simulink model "RobotX_ss_acousticsSingle_Dock_LBskip_ODOA_T_1024_NewLidarMode"  (R2014a)
settings: Solver=FixedStepDiscrete  StartTime=0.0  StopTime=inf  FixedStep=.25  RelTol=1e-3
undefined symbols (not defined in the file): Com1, Com2, Com3, Com4, DiscIntNeverNeededParam, standard
libraries: xpcseriallib x42, simulink x19, slrtlib x7, dspmtrx3 x2, speedgoatlib x2, speedgoatlib_IO102 x1
(part 3 of 7)

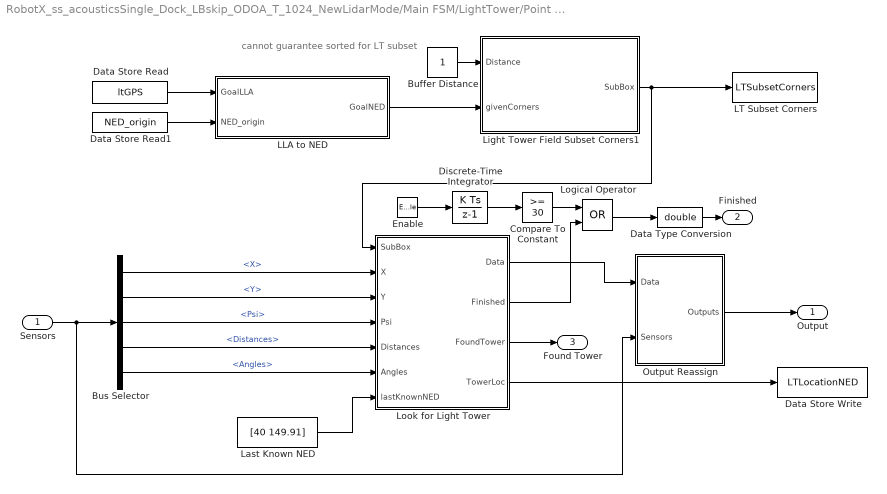
== system RobotX_ss_acousticsSingle_Dock_LBskip_ODOA_T_1024_NewLidarMode/Main FSM/LightTower/Point Toward Last Known Heading ==
  note: cannot guarantee sorted for LT subset
  Sensors : Inport
  Enable : EnablePort  ShowOutputPort=on
  Buffer Distance : Constant
  Bus Selector : BusSelector  OutputSignals=Navigation Message.Pose.X,Navigation Message.Pose.Y,Navigation Message.Pose.Psi,Lidar Data Input.Landmarks.Distances,Lidar Data Input.Landmarks.Angles
  Compare To Constant : simulink/Logic and Bit Operations/Compare To Constant  relop=>=  const=30  OutDataTypeStr=boolean
  Data Store Read : DataStoreRead  DataStoreName=ltGPS
  Data Store Read1 : DataStoreRead  DataStoreName=NED_origin
  Data Store Write : DataStoreWrite  DialogController=Simulink.DDGSource  DataStoreName=LTLocationNED
  Data Type Conversion : DataTypeConversion  OutDataTypeStr=double
  Discrete-Time Integrator : DiscreteIntegrator  SampleTime=-1  ICPrevOutput=DiscIntNeverNeededParam  ICPrevScaledInput=DiscIntNeverNeededParam
  LLA to NED : MATLAB Function  TreatAsAtomicUnit=on
  LT Subset Corners : DataStoreWrite  DataStoreName=LTSubsetCorners
  Last Known NED : Constant  Value=[40 149.91]
  Light Tower Field Subset Corners1 : MATLAB Function  TreatAsAtomicUnit=on
  Logical Operator : Logic  Operator=OR  AllPortsSameDT=off  OutDataTypeStr=boolean
  Look for Light Tower : MATLAB Function  TreatAsAtomicUnit=on
  Output Reassign : Subsystem
  Output : Outport
  Finished : Outport  Port=2
  Found Tower : Outport  Port=3
  wires:
  Output Reassign/1(Outputs) -> Output/1
  Sensors/1 -> Output Reassign/2(Sensors), Bus Selector/1
  Data Store Read/1 -> LLA to NED/1(GoalLLA)
  Data Store Read1/1 -> LLA to NED/2(NED_origin)
  LLA to NED/1(GoalNED) -> Light Tower Field Subset Corners1/2(givenCorners)
  Buffer Distance/1 -> Light Tower Field Subset Corners1/1(Distance)
  Bus Selector/1 -> Look for Light Tower/2(X)  "<X>"
  Bus Selector/2 -> Look for Light Tower/3(Y)  "<Y>"
  Bus Selector/3 -> Look for Light Tower/4(Psi)  "<Psi>"
  Bus Selector/4 -> Look for Light Tower/5(Distances)  "<Distances>"
  Bus Selector/5 -> Look for Light Tower/6(Angles)  "<Angles>"
  Light Tower Field Subset Corners1/1(SubBox) -> Look for Light Tower/1(SubBox), LT Subset Corners/1
  Look for Light Tower/1(Data) -> Output Reassign/1(Data)
  Look for Light Tower/2(Finished) -> Logical Operator/2
  Look for Light Tower/3(FoundTower) -> Found Tower/1
  Last Known NED/1 -> Look for Light Tower/7(lastKnownNED)
  Look for Light Tower/4(TowerLoc) -> Data Store Write/1
  Enable/1 -> Discrete-Time Integrator/1
  Discrete-Time Integrator/1 -> Compare To Constant/1
  Compare To Constant/1 -> Logical Operator/1
  Logical Operator/1 -> Data Type Conversion/1
  Data Type Conversion/1 -> Finished/1

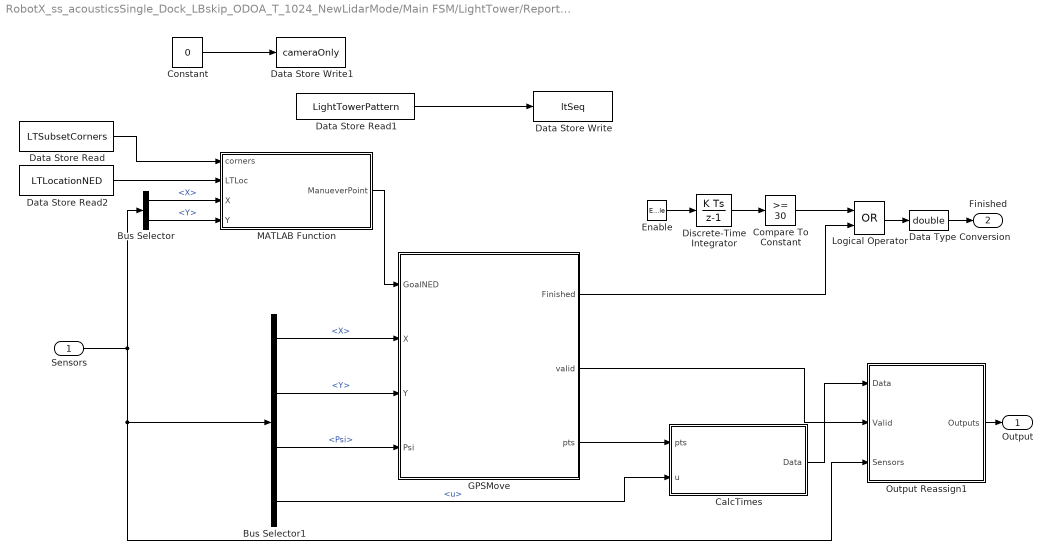
== system RobotX_ss_acousticsSingle_Dock_LBskip_ODOA_T_1024_NewLidarMode/Main FSM/LightTower/Report and Manuever Away ==
  Sensors : Inport
  Enable : EnablePort  ShowOutputPort=on
  Bus Selector : BusSelector  OutputSignals=Navigation Message.Pose.X,Navigation Message.Pose.Y
  Bus Selector1 : BusSelector  OutputSignals=Navigation Message.Pose.X,Navigation Message.Pose.Y,Navigation Message.Pose.Psi,Navigation Message.Velocity.u
  CalcTimes : MATLAB Function  TreatAsAtomicUnit=on
  Compare To Constant : simulink/Logic and Bit Operations/Compare To Constant  relop=>=  const=30  OutDataTypeStr=boolean
  Constant : Constant  Value=0
  Data Store Read : DataStoreRead  DataStoreName=LTSubsetCorners
  Data Store Read1 : DataStoreRead  DialogController=Simulink.DDGSource  DataStoreName=LightTowerPattern
  Data Store Read2 : DataStoreRead  DialogController=Simulink.DDGSource  DataStoreName=LTLocationNED
  Data Store Write : DataStoreWrite  DialogController=Simulink.DDGSource  DataStoreName=ltSeq
  Data Store Write1 : DataStoreWrite  DataStoreName=cameraOnly
  Data Type Conversion : DataTypeConversion  OutDataTypeStr=double
  Discrete-Time Integrator : DiscreteIntegrator  SampleTime=-1  ICPrevOutput=DiscIntNeverNeededParam  ICPrevScaledInput=DiscIntNeverNeededParam
  GPSMove : MATLAB Function  TreatAsAtomicUnit=on
  Logical Operator : Logic  Operator=OR  AllPortsSameDT=off  OutDataTypeStr=boolean
  MATLAB Function : MATLAB Function  TreatAsAtomicUnit=on
  Output Reassign1 : Subsystem
  Output : Outport
  Finished : Outport  Port=2
  wires:
  Output Reassign1/1(Outputs) -> Output/1
  Data Store Read/1 -> MATLAB Function/1(corners)
  Sensors/1 -> Bus Selector/1, Output Reassign1/3(Sensors), Bus Selector1/1
  Bus Selector/1 -> MATLAB Function/3(X)  "<X>"
  Bus Selector/2 -> MATLAB Function/4(Y)  "<Y>"
  GPSMove/1(Finished) -> Logical Operator/2
  GPSMove/3(pts) -> CalcTimes/1(pts)
  Bus Selector1/1 -> GPSMove/2(X)  "<X>"
  Bus Selector1/2 -> GPSMove/3(Y)  "<Y>"
  Bus Selector1/3 -> GPSMove/4(Psi)  "<Psi>"
  Bus Selector1/4 -> CalcTimes/2(u)  "<u>"
  CalcTimes/1(Data) -> Output Reassign1/1(Data)
  GPSMove/2(valid) -> Output Reassign1/2(Valid)
  MATLAB Function/1(ManueverPoint) -> GPSMove/1(GoalNED)
  Data Store Read1/1 -> Data Store Write/1
  Data Store Read2/1 -> MATLAB Function/2(LTLoc)
  Discrete-Time Integrator/1 -> Compare To Constant/1
  Enable/1 -> Discrete-Time Integrator/1
  Compare To Constant/1 -> Logical Operator/1
  Logical Operator/1 -> Data Type Conversion/1
  Data Type Conversion/1 -> Finished/1
  Constant/1 -> Data Store Write1/1

== system RobotX_ss_acousticsSingle_Dock_LBskip_ODOA_T_1024_NewLidarMode/Main FSM/LightTower/Sweep Field ==
  Sensors : Inport
  Enable : EnablePort  ShowOutputPort=on
  Bus Creator : BusCreator  Inputs=2
  Bus Selector : BusSelector  OutputSignals=Drive to Point Fin,Spin & Listen Fin
  Compare To Constant : simulink/Logic and Bit Operations/Compare To Constant  relop=>=  const=30  OutDataTypeStr=boolean
  Data Type Conversion : DataTypeConversion  OutDataTypeStr=double
  Discrete-Time Integrator : DiscreteIntegrator  SampleTime=-1  ICPrevOutput=DiscIntNeverNeededParam  ICPrevScaledInput=DiscIntNeverNeededParam
  Drive to Point : Subsystem
  Logical Operator : Logic  Operator=OR  Inputs=3  AllPortsSameDT=off  OutDataTypeStr=boolean
  Multiport Switch : MultiPortSwitch  Inputs=2
  "Spin, Listen, and Point" : Subsystem
  Sweep Field Enabler : MATLAB Function  TreatAsAtomicUnit=on
  Task Option : Subsystem
  Unit Delay : UnitDelay  SampleTime=-1
  Outputs : Outport
  Finished : Outport  Port=2
  wires:
  Drive to Point/1(Outputs) -> Multiport Switch/2
  "Spin, Listen, and Point"/1(Outputs) -> Multiport Switch/3
  Multiport Switch/1 -> Outputs/1
  Data Type Conversion/1 -> Finished/1
  Sensors/1 -> "Spin, Listen, and Point"/1(Sensors), Drive to Point/1(Sensors)
  Task Option/1(Option) -> Sweep Field Enabler/1(Sweep)
  "Spin, Listen, and Point"/2(Finished) -> Bus Creator/2  "Spin & Listen Fin"
  Sweep Field Enabler/2(drivePointEn) -> Drive to Point/Enable
  Sweep Field Enabler/1(taskSelector) -> Multiport Switch/1
  Sweep Field Enabler/3(spinListenEn) -> "Spin, Listen, and Point"/Enable
  Drive to Point/2(Finished) -> Bus Creator/1  "Drive to Point Fin"
  Bus Creator/1 -> Unit Delay/1
  "Spin, Listen, and Point"/3(Found LT) -> Logical Operator/2
  Unit Delay/1 -> Bus Selector/1
  Bus Selector/1 -> Sweep Field Enabler/2(drivePointFin)  "<Drive to Point Fin>"
  Bus Selector/2 -> Sweep Field Enabler/3(spinFin)  "<Spin & Listen Fin>"
  Drive to Point/3(Found LT) -> Logical Operator/1
  Logical Operator/1 -> Data Type Conversion/1
  Discrete-Time Integrator/1 -> Compare To Constant/1
  Enable/1 -> Discrete-Time Integrator/1
  Compare To Constant/1 -> Logical Operator/3

== system RobotX_ss_acousticsSingle_Dock_LBskip_ODOA_T_1024_NewLidarMode/Main FSM/LightTower/Turn For Approach1  ==
  note: Signal
  Sensors : Inport
  Enable : EnablePort  ShowOutputPort=on
  Bus Selector : BusSelector  OutputSignals=Navigation Message.Pose.X,Navigation Message.Pose.Y
  Compare To Constant : simulink/Logic and Bit Operations/Compare To Constant  relop=>=  const=30  OutDataTypeStr=boolean
  Data Type Conversion : DataTypeConversion  OutDataTypeStr=double
  Discrete-Time Integrator : DiscreteIntegrator  SampleTime=-1  ICPrevOutput=DiscIntNeverNeededParam  ICPrevScaledInput=DiscIntNeverNeededParam
  LTLoc : DataStoreRead  DialogController=Simulink.DDGSource  DataStoreName=LTLocationNED
  MATLAB1 Function : MATLAB Function  TreatAsAtomicUnit=on
  Output Heirarchy : Subsystem
  Outputs : Outport
  Finished : Outport  Port=2
  wires:
  Discrete-Time Integrator/1 -> Compare To Constant/1
  Enable/1 -> Discrete-Time Integrator/1
  Compare To Constant/1 -> Data Type Conversion/1
  Data Type Conversion/1 -> Finished/1
  Sensors/1 -> Bus Selector/1, Output Heirarchy/2(Sensors)
  MATLAB1 Function/1(Data) -> Output Heirarchy/1(Data)
  Output Heirarchy/1(Outputs) -> Outputs/1
  Bus Selector/2 -> MATLAB1 Function/3(Y)  "<Y>"
  Bus Selector/1 -> MATLAB1 Function/2(X)  "<X>"
  LTLoc/1 -> MATLAB1 Function/1(LTLoc)

== system RobotX_ss_acousticsSingle_Dock_LBskip_ODOA_T_1024_NewLidarMode/Main FSM/LightTower/Turn For Sweep ==
  note: Signal
  Sensors : Inport
  Enable : EnablePort  ShowOutputPort=on
  Bus Selector : BusSelector  OutputSignals=Navigation Message.Pose.X,Navigation Message.Pose.Y
  Compare To Constant : simulink/Logic and Bit Operations/Compare To Constant  relop=>=  const=30  OutDataTypeStr=boolean
  Data Store Read : DataStoreRead  DataStoreName=ltGPS
  Data Store Read1 : DataStoreRead  DataStoreName=NED_origin
  Data Type Conversion : DataTypeConversion  OutDataTypeStr=double
  Discrete-Time Integrator : DiscreteIntegrator  SampleTime=-1  ICPrevOutput=DiscIntNeverNeededParam  ICPrevScaledInput=DiscIntNeverNeededParam
  LLA to NED : MATLAB Function  TreatAsAtomicUnit=on
  MATLAB Function : MATLAB Function  TreatAsAtomicUnit=on
  Output Heirarchy : Subsystem
  Outputs : Outport
  Finished : Outport  Port=2
  wires:
  Discrete-Time Integrator/1 -> Compare To Constant/1
  Enable/1 -> Discrete-Time Integrator/1
  Compare To Constant/1 -> Data Type Conversion/1
  Data Type Conversion/1 -> Finished/1
  Sensors/1 -> Bus Selector/1, Output Heirarchy/2(Sensors)
  MATLAB Function/1(Data) -> Output Heirarchy/1(Data)
  Output Heirarchy/1(Outputs) -> Outputs/1
  Bus Selector/2 -> MATLAB Function/3(Y)  "<Y>"
  Bus Selector/1 -> MATLAB Function/2(X)  "<X>"
  Data Store Read/1 -> LLA to NED/1(GoalLLA)
  Data Store Read1/1 -> LLA to NED/2(NED_origin)
  LLA to NED/1(GoalNED) -> MATLAB Function/1(ltPTS)

== system RobotX_ss_acousticsSingle_Dock_LBskip_ODOA_T_1024_NewLidarMode/Main FSM/LightTower/Wait for Sequence ==
  Sensors : Inport
  Enable : EnablePort  ShowOutputPort=on
  Bus Selector1 : BusSelector  OutputSignals=Lidar Data Input.Color data.Color
  Constant : Constant
  Data Store Read : DataStoreRead  DataStoreName=holdPose
  Data Store Write : DataStoreWrite  DataStoreName=LightTowerPattern
  Data Store Write1 : DataStoreWrite  DataStoreName=cameraOnly
  Discrete-Time Integrator : DiscreteIntegrator  SampleTime=-1  ICPrevOutput=DiscIntNeverNeededParam  ICPrevScaledInput=DiscIntNeverNeededParam
  MATLAB Function : MATLAB Function  TreatAsAtomicUnit=on
  MATLAB Function1 : MATLAB Function  TreatAsAtomicUnit=on
  Output Reassign1 : Subsystem
  Output : Outport
  Finished : Outport  Port=2
  wires:
  Sensors/1 -> Bus Selector1/1, Output Reassign1/2(Sensors)
  Output Reassign1/1(Outputs) -> Output/1
  MATLAB Function/1(Data) -> Output Reassign1/1(Data)
  MATLAB Function1/2(Pattern) -> Data Store Write/1
  Bus Selector1/1 -> MATLAB Function1/2(visionData)  "<Color>"
  Enable/1 -> Discrete-Time Integrator/1
  Discrete-Time Integrator/1 -> MATLAB Function1/1(time)
  MATLAB Function1/1(Finished) -> Finished/1
  Data Store Read/1 -> MATLAB Function/1(holdPose)
  Constant/1 -> Data Store Write1/1

== system RobotX_ss_acousticsSingle_Dock_LBskip_ODOA_T_1024_NewLidarMode/Main FSM/ODOA/Dodge ==
  Sensors : Inport
  Enable : EnablePort  ShowOutputPort=on
  Bus Selector : BusSelector  OutputSignals=Navigation Message.Pose.X,Navigation Message.Pose.Y,Navigation Message.Pose.Psi,Lidar Data Input.Landmarks.Distances,Lidar Data Input.Landmarks.Angles,Navigation Message.Velocity.u
  CalcTimes : MATLAB Function  TreatAsAtomicUnit=on
  Constant : Constant  Value=0
  Data Store Write : DataStoreWrite  DataStoreName=dodgeStart
  Discrete-Time Integrator : DiscreteIntegrator  SampleTime=-1  ICPrevOutput=DiscIntNeverNeededParam  ICPrevScaledInput=DiscIntNeverNeededParam
  Dodge : MATLAB Function  TreatAsAtomicUnit=on
  Nav Logic : MATLAB Function  Commented=on  TreatAsAtomicUnit=on
  Output Reassign : Subsystem
  Unit Delay1 : UnitDelay  InitialCondition=1  SampleTime=-1
  Outputs : Outport
  Dodge Incomplete : Outport  Port=2
  wires:
  Sensors/1 -> Output Reassign/3(Sensors), Bus Selector/1
  Enable/1 -> Discrete-Time Integrator/1
  Discrete-Time Integrator/1 -> Dodge/1(time)
  Constant/1 -> Unit Delay1/1
  Unit Delay1/1 -> Data Store Write/1
  Output Reassign/1(Outputs) -> Outputs/1
  Bus Selector/3 -> Dodge/4(Psi)  "<Psi>"
  Bus Selector/5 -> Dodge/6(Angles)  "<Angles>"
  Bus Selector/1 -> Dodge/2(X)  "<X>"
  Bus Selector/2 -> Dodge/3(Y)  "<Y>"
  Bus Selector/4 -> Dodge/5(Dist)  "<Distances>"
  Dodge/3(pts) -> CalcTimes/1(pts)
  Bus Selector/6 -> CalcTimes/2(u)  "<u>"
  Dodge/2(Valid) -> Output Reassign/1(Vaild)
  CalcTimes/1(Data) -> Output Reassign/2(Data)
  Dodge/1(dodgeIncomplete) -> Dodge Incomplete/1

== system RobotX_ss_acousticsSingle_Dock_LBskip_ODOA_T_1024_NewLidarMode/Main FSM/ODOA/Entry Gate ==
  Sensors : Inport
  Enable : EnablePort
  Bus Creator : BusCreator  Inputs=2
  Bus Selector : BusSelector  OutputSignals=Start Fin,Align Fin
  Entry Gate Align : Subsystem  TreatAsAtomicUnit=on
  Entry Gate Enabler : MATLAB Function  TreatAsAtomicUnit=on
  Entry Gate Through : Subsystem
  GPS Move : Subsystem
  Multiport Switch : MultiPortSwitch
  Unit Delay : UnitDelay  SampleTime=-1
  Outputs : Outport
  Finished : Outport  Port=2
  wires:
  Multiport Switch/1 -> Outputs/1
  Entry Gate Enabler/3(AlignEn) -> Entry Gate Align/Enable
  Sensors/1 -> GPS Move/1(Sensors), Entry Gate Through/1(Sensors), Entry Gate Align/1(Sensors)
  Entry Gate Through/2(Finished) -> Finished/1
  Entry Gate Enabler/4(ThroughEn) -> Entry Gate Through/Enable
  Unit Delay/1 -> Bus Selector/1
  Entry Gate Through/1(Outputs) -> Multiport Switch/4
  Entry Gate Enabler/1(TaskSelector) -> Multiport Switch/1
  Entry Gate Enabler/2(StartEn) -> GPS Move/Enable
  GPS Move/2(Finished) -> Bus Creator/1  "Start Fin"
  Entry Gate Align/2(Finished) -> Bus Creator/2  "Align Fin"
  Entry Gate Align/1(Outputs) -> Multiport Switch/3
  GPS Move/1(Outputs) -> Multiport Switch/2
  Bus Creator/1 -> Unit Delay/1
  Bus Selector/2 -> Entry Gate Enabler/2(AlignFin)  "<Align Fin>"
  Bus Selector/1 -> Entry Gate Enabler/1(StartFin)  "<Start Fin>"

== system RobotX_ss_acousticsSingle_Dock_LBskip_ODOA_T_1024_NewLidarMode/Main FSM/ODOA/Exit Gate ==
  Sensors : Inport
  Enable : EnablePort
  Exit Gate Align : Subsystem  TreatAsAtomicUnit=on
  Exit Gate Through : Subsystem
  Multiport Switch : MultiPortSwitch  Inputs=2
  Unit Delay : UnitDelay  SampleTime=-1
  exit Gate Enabler : MATLAB Function  TreatAsAtomicUnit=on
  Outputs : Outport
  Finished : Outport  Port=2
  wires:
  Multiport Switch/1 -> Outputs/1
  exit Gate Enabler/2(AlignEn) -> Exit Gate Align/Enable
  Sensors/1 -> Exit Gate Through/1(Sensors), Exit Gate Align/1(Sensors)
  Exit Gate Through/2(Finished) -> Finished/1
  exit Gate Enabler/3(ThroughEn) -> Exit Gate Through/Enable
  Exit Gate Through/1(Outputs) -> Multiport Switch/3
  exit Gate Enabler/1(TaskSelector) -> Multiport Switch/1
  Exit Gate Align/2(Finished) -> Unit Delay/1  "Align Fin"
  Exit Gate Align/1(Outputs) -> Multiport Switch/2
  Unit Delay/1 -> exit Gate Enabler/1(AlignFin)

== system RobotX_ss_acousticsSingle_Dock_LBskip_ODOA_T_1024_NewLidarMode/Main FSM/ODOA/GPS Beeline ==
  Sensors : Inport
  Enable : EnablePort
  Bus Selector : BusSelector  OutputSignals=Navigation Message.Pose.X,Navigation Message.Pose.Y,Navigation Message.Pose.Psi,Lidar Data Input.Landmarks.Distances,Navigation Message.Velocity.u
  CalcTimes : MATLAB Function  TreatAsAtomicUnit=on
  Data Store Read : DataStoreRead  DataStoreName=ExitGateNED
  Data Store Read1 : DataStoreRead  DataStoreName=ODOAexit
  Data Store Write : DataStoreWrite  DataStoreName=dodgeStart
  GPSMove : MATLAB Function  TreatAsAtomicUnit=on
  MATLAB Function1 : MATLAB Function  TreatAsAtomicUnit=on
  Output Reassign : Subsystem
  Unit Delay1 : UnitDelay  SampleTime=-1
  Outputs : Outport
  Finished : Outport  Port=2
  wires:
  GPSMove/4(pts) -> CalcTimes/1(pts)
  Sensors/1 -> Output Reassign/3(Sensors), Bus Selector/1
  Bus Selector/1 -> GPSMove/2(X)  "<X>"
  Bus Selector/2 -> GPSMove/3(Y)  "<Y>"
  Bus Selector/3 -> GPSMove/4(Psi)  "<Psi>"
  Bus Selector/5 -> CalcTimes/2(u)  "<u>"
  GPSMove/2(Finished) -> Finished/1
  Output Reassign/1(Outputs) -> Outputs/1
  CalcTimes/1(Data) -> Output Reassign/2(Data)
  GPSMove/3(valid) -> Output Reassign/1(Vaild)
  MATLAB Function1/1(exitGPS) -> GPSMove/1(GoalNED)
  Data Store Read1/1 -> MATLAB Function1/2(gateNumber)
  Data Store Read/1 -> MATLAB Function1/1(ExitGateGPS)
  Unit Delay1/1 -> Data Store Write/1
  Bus Selector/4 -> GPSMove/5(Distances)  "<Distances>"
  GPSMove/1(dodgeStart) -> Unit Delay1/1

== system RobotX_ss_acousticsSingle_Dock_LBskip_ODOA_T_1024_NewLidarMode/Main FSM/RCHold/Direct Control ==
  Sensors : Inport
  Acoustic Active : Constant  Value=0
  Bus Creator2 : BusCreator  Inputs=3
  Bus Creator3 : BusCreator  Inputs=3
  Bus Creator4 : BusCreator  Inputs=2
  Constant : Constant
  Constant1 : Constant  Value=2
  Constant2 : Constant  Value=zeros(24,1)
  Lidar Mode : Constant  Value=3
  Outputs : Outport
  wires:
  Sensors/1 -> Bus Creator4/2  "Sensors"
  Bus Creator4/1 -> Outputs/1  "Output Signals"
  Bus Creator2/1 -> Bus Creator3/1  "Navigation Outputs"
  Acoustic Active/1 -> Bus Creator3/2  "Acoustic Active"
  Lidar Mode/1 -> Bus Creator3/3  "Lidar Mode"
  Bus Creator3/1 -> Bus Creator4/1  "Outputs"
  Constant/1 -> Bus Creator2/1  "Valid"
  Constant1/1 -> Bus Creator2/2  "Control Mode"
  Constant2/1 -> Bus Creator2/3  "Data"

== system RobotX_ss_acousticsSingle_Dock_LBskip_ODOA_T_1024_NewLidarMode/Main FSM/Start//Speedgate/Aim ==
  note: Signal
  Sensors : Inport
  Enable : EnablePort  ShowOutputPort=on
  Compare To Constant : simulink/Logic and Bit Operations/Compare To Constant  relop=>=  const=30  OutDataTypeStr=boolean
  Data Store Read : DataStoreRead  DataStoreName=ssHeldHeading
  Data Store Read1 : DataStoreRead  Commented=on  DataStoreName=startGPS
  Data Store Read2 : DataStoreRead  Commented=on  DataStoreName=NED_origin
  Data Store Read3 : DataStoreRead  DataStoreName=startNED
  Data Type Conversion : DataTypeConversion  OutDataTypeStr=double
  Discrete-Time Integrator : DiscreteIntegrator  SampleTime=-1  ICPrevOutput=DiscIntNeverNeededParam  ICPrevScaledInput=DiscIntNeverNeededParam
  LLA to NED : MATLAB Function  Commented=on  TreatAsAtomicUnit=on
  MATLAB Function : MATLAB Function  TreatAsAtomicUnit=on
  Output Heirarchy : Subsystem
  Outputs : Outport
  Finished : Outport  Port=2
  wires:
  Discrete-Time Integrator/1 -> Compare To Constant/1
  Enable/1 -> Discrete-Time Integrator/1
  Compare To Constant/1 -> Data Type Conversion/1
  Data Type Conversion/1 -> Finished/1
  Sensors/1 -> Output Heirarchy/2(Sensors)
  MATLAB Function/1(Data) -> Output Heirarchy/1(Data)
  Output Heirarchy/1(Outputs) -> Outputs/1
  Data Store Read/1 -> MATLAB Function/1(ssHeldHeading)
  LLA to NED/1(GoalNED) -> ?
  Data Store Read2/1 -> LLA to NED/2(NED_origin)
  Data Store Read1/1 -> LLA to NED/1(LLA)
  Data Store Read3/1 -> MATLAB Function/2(ssGateNED)

== system RobotX_ss_acousticsSingle_Dock_LBskip_ODOA_T_1024_NewLidarMode/Main FSM/Start//Speedgate/Dead Reckon ==
  note: Through Gate
  Sensors : Inport
  Enable : EnablePort
  Bus Selector : BusSelector  OutputSignals=Navigation Message.Pose.X,Navigation Message.Pose.Y,Navigation Message.Velocity.u
  Calculate Times : MATLAB Function  TreatAsAtomicUnit=on
  Data Store Read : DataStoreRead  DataStoreName=ssHeldHeading
  Gate : MATLAB Function  TreatAsAtomicUnit=on
  Output Reassign : Subsystem
  sglength : Constant  Value=15
  Outputs : Outport
  Finished : Outport  Port=2
  wires:
  Output Reassign/1(Outputs) -> Outputs/1
  Gate/1(Finished) -> Finished/1
  Sensors/1 -> Output Reassign/3(Sensors), Bus Selector/1
  Bus Selector/2 -> Gate/4(Y)  "<Y>"
  Bus Selector/1 -> Gate/3(X)  "<X>"
  Bus Selector/3 -> Calculate Times/2(u)  "<u>"
  Gate/3(pts) -> Calculate Times/1(pts)
  Calculate Times/1(Data) -> Output Reassign/2(Data)
  Gate/2(Valid) -> Output Reassign/1(Vaild)
  Data Store Read/1 -> Gate/2(ssHeldHeading)
  sglength/1 -> Gate/1(sglength)

== system RobotX_ss_acousticsSingle_Dock_LBskip_ODOA_T_1024_NewLidarMode/Main FSM/Start//Speedgate/GPS Move ==
  Sensors : Inport
  Enable : EnablePort
  Bus Selector : BusSelector  OutputSignals=Navigation Message.Pose.X,Navigation Message.Pose.Y,Navigation Message.Pose.Psi,Navigation Message.Velocity.u
  CalcTimes : MATLAB Function  TreatAsAtomicUnit=on
  Data Store Read1 : DataStoreRead  Commented=on  DataStoreName=startGPS
  Data Store Read2 : DataStoreRead  Commented=on  DataStoreName=NED_origin
  Data Store Read3 : DataStoreRead  DataStoreName=startNED
  GPSMove : MATLAB Function  TreatAsAtomicUnit=on
  LLA to NED : MATLAB Function  Commented=on  TreatAsAtomicUnit=on
  Output Reassign : Subsystem
  Outputs : Outport
  Finished : Outport  Port=2
  wires:
  GPSMove/3(pts) -> CalcTimes/1(pts)
  Sensors/1 -> Output Reassign/3(Sensors), Bus Selector/1
  Bus Selector/1 -> GPSMove/2(X)  "<X>"
  Bus Selector/2 -> GPSMove/3(Y)  "<Y>"
  Bus Selector/3 -> GPSMove/4(Psi)  "<Psi>"
  Bus Selector/4 -> CalcTimes/2(u)  "<u>"
  GPSMove/1(Finished) -> Finished/1
  Output Reassign/1(Outputs) -> Outputs/1
  CalcTimes/1(Data) -> Output Reassign/2(Data)
  GPSMove/2(valid) -> Output Reassign/1(Vaild)
  LLA to NED/1(GoalNED) -> ?
  Data Store Read3/1 -> GPSMove/1(GoalNED)
  Data Store Read2/1 -> LLA to NED/2(NED_origin)
  Data Store Read1/1 -> LLA to NED/1(LLA)

== system RobotX_ss_acousticsSingle_Dock_LBskip_ODOA_T_1024_NewLidarMode/Main FSM/Termination/Output Reassign ==
  Vaild : Inport
  Data : Inport  Port=2
  Sensors : Inport  Port=3
  Acoustic Active : Constant  Value=0
  Bus Creator2 : BusCreator  Inputs=3
  Bus Creator3 : BusCreator  Inputs=3
  Bus Creator5 : BusCreator  Inputs=2
  Constant3 : Constant  Value=0
  Lidar Mode : Constant  Value=0
  Outputs : Outport
  wires:
  Sensors/1 -> Bus Creator5/2  "Sensors"
  Bus Creator5/1 -> Outputs/1  "Output Signals"
  Vaild/1 -> Bus Creator2/1  "Valid"
  Constant3/1 -> Bus Creator2/2  "Control Mode"
  Data/1 -> Bus Creator2/3  "Data"
  Bus Creator2/1 -> Bus Creator3/1  "Navigation Outputs"
  Acoustic Active/1 -> Bus Creator3/2  "Acoustic Active"
  Lidar Mode/1 -> Bus Creator3/3  "Lidar Mode"
  Bus Creator3/1 -> Bus Creator5/1  "Outputs"

== system RobotX_ss_acousticsSingle_Dock_LBskip_ODOA_T_1024_NewLidarMode/Sensors/1020 Comms/ Raspberry Pi LCM (Acoustic) ==
  LCM Input : Inport
  ASCII Decode 6 : xpcseriallib/ASCII Decode   format=Deploy:%1u, Elapsed:%g, Bearing1:%g Bearing2:%g \r\n  nvars=4  vartypes={}
  Bus Creator : BusCreator  Inputs=2
  Bus Creator1 : BusCreator  Inputs=3
  FIFO ASCII read 1 : xpcseriallib/FIFO ASCII read   header={'Deploy:'}  term=[13 10]  hold=Zero output if no new data  enable=off  maxsize=1024  outputtype=8 bit uint null terminated  sampletime=-1
  LCM Output : Outport
  wires:
  LCM Input/1 -> FIFO ASCII read 1/1
  FIFO ASCII read 1/1 -> ASCII Decode 6/1
  ASCII Decode 6/3 -> Bus Creator/1  "Horizontal Bearing"
  ASCII Decode 6/4 -> Bus Creator/2  "Vertical Bearing"
  Bus Creator/1 -> Bus Creator1/3  "Bearings"
  ASCII Decode 6/2 -> Bus Creator1/2  "Elapsed Time"
  ASCII Decode 6/1 -> Bus Creator1/1  "Deployed"
  Bus Creator1/1 -> LCM Output/1  "Acoustic Message"

== system RobotX_ss_acousticsSingle_Dock_LBskip_ODOA_T_1024_NewLidarMode/Sensors/1020 Comms/ Raspberry Pi LCM (Navigation and Acoustics) ==
  LCM Input : Inport
  ASCII Decode 6 : xpcseriallib/ASCII Decode   format=P1:%f P2:%f P3:%f V1:%f V2:%f V3:%f E1:%f E2:%f E3:%f Pt1:%f Pt2:%f St1:%f St2:%f Start:%f Elapsed:%f RC:%d Deploy:%u, Elapsed:%g, Bearing1:%g Bearing2:%g \r\n  nvars=22  vartypes={}
  Bus Creator{,5..7} (4 alike) : BusCreator  Inputs=2
  Bus Creator{1..3,8} (4 alike) : BusCreator  Inputs=3
  Bus Creator4 : BusCreator  Inputs=9
  Data Type Conversion : DataTypeConversion  OutDataTypeStr=double
  FIFO ASCII read 1 : xpcseriallib/FIFO ASCII read   header={'P1:'}  term=[13 10]  hold=Zero output if no new data  enable=off  maxsize=2048  outputtype=8 bit uint null terminated  sampletime=-1
  Navigation LCM : Outport
  Acoustic LCM : Outport  Port=2
  wires:
  LCM Input/1 -> FIFO ASCII read 1/1
  FIFO ASCII read 1/1 -> ASCII Decode 6/1
  Bus Creator4/1 -> Navigation LCM/1  "Navigation Message"
  ASCII Decode 6/1 -> Bus Creator1/1  "X"
  ASCII Decode 6/2 -> Bus Creator1/2  "Y"
  ASCII Decode 6/3 -> Bus Creator1/3  "Psi"
  Bus Creator1/1 -> Bus Creator4/1  "Pose"
  ASCII Decode 6/4 -> Bus Creator2/1  "u"
  ASCII Decode 6/5 -> Bus Creator2/2  "v"
  Bus Creator2/1 -> Bus Creator4/2  "Velocity"
  ASCII Decode 6/7 -> Bus Creator3/1  "Roll"
  ASCII Decode 6/8 -> Bus Creator3/2  "Pitch"
  ASCII Decode 6/9 -> Bus Creator3/3  "Yaw"
  Bus Creator3/1 -> Bus Creator4/3  "Euler"
  Bus Creator5/1 -> Bus Creator4/5  "Port"
  Bus Creator6/1 -> Bus Creator4/6  "Stbd"
  ASCII Decode 6/14 -> Bus Creator6/1  "StThrust"
  ASCII Decode 6/15 -> Bus Creator6/2  "StAzimuth"
  ASCII Decode 6/12 -> Bus Creator5/1  "PtThrust"
  ASCII Decode 6/13 -> Bus Creator5/2  "PtAzimuth"
  ASCII Decode 6/16 -> Bus Creator4/7  "Start"
  ASCII Decode 6/17 -> Bus Creator4/8  "Elapsed"
  ASCII Decode 6/18 -> Data Type Conversion/1  "On/Off/RC/Auto"
  Data Type Conversion/1 -> Bus Creator4/9  "On/Off/RC/Auto"
  ASCII Decode 6/6 -> Bus Creator2/3  "r"
  ASCII Decode 6/10 -> Bus Creator7/1  "Lat"
  ASCII Decode 6/11 -> Bus Creator7/2  "Long"
  Bus Creator7/1 -> Bus Creator4/4  "GPS (LLA)"
  ASCII Decode 6/21 -> Bus Creator/1  "Horizontal Bearing"
  ASCII Decode 6/22 -> Bus Creator/2  "Vertical Bearing"
  Bus Creator/1 -> Bus Creator8/3  "Bearings"
  ASCII Decode 6/20 -> Bus Creator8/2  "Elapsed Time"
  ASCII Decode 6/19 -> Bus Creator8/1  "Deployed"
  Bus Creator8/1 -> Acoustic LCM/1  "Acoustic Message"

== matlab function RobotX_ss_acousticsSingle_Dock_LBskip_ODOA_T_1024_NewLidarMode/Main FSM/Acoustic Single Point FSM/Move/GPSMove ==
  data: GoalNED input; X input; Finished output; valid output; Y input; Psi input; pts output
function [Finished,valid,pts] = GPSmove(GoalNED,X,Y,Psi)
%Written by Dylan DeGaetano on September 1, 2014
%Last edited by: Anderson Lebbad
%
%This function will go to a given NED cooridnate, last edit changed the
%goal pt and variable names

persistent Sample
if isempty(Sample)
Sample = 0;
end
Finished = 0;
pts = zeros(8,2);
%$Distance to object in meters
if Sample >= 100
    Sample = 0;
end

if Sample == 0
    pts(1,1) = X+5*cos(Psi*pi/180);
    pts(1,2) = Y+5*sin(Psi*pi/180);
    pts(8,1) = GoalNED(1,1);
    pts(8,2) = GoalNED(1,2);
    pts(2,:) = pts(1,:) +(1*(GoalNED-pts(1,:))/7);
    pts(3,:) = pts(1,:) +(2*(GoalNED-pts(1,:))/7);
    pts(4,:) = pts(1,:) +(3*(GoalNED-pts(1,:))/7);
    pts(5,:) = pts(1,:) +(4*(GoalNED-pts(1,:))/7);
    pts(6,:) = pts(1,:) +(5*(GoalNED-pts(1,:))/7);
    pts(7,:) = pts(1,:) +(6*(GoalNED-pts(1,:))/7);
    Sample = 1; 
    valid = 1;
    
else 
    range = sqrt(sum((GoalNED - [X Y]).^2));
    if range <= 5
        Finished = 1;
    end
    valid = 0;
    Sample = Sample + 1;
end

== matlab function RobotX_ss_acousticsSingle_Dock_LBskip_ODOA_T_1024_NewLidarMode/Main FSM/LightTower/Point Toward Last Known Heading/LLA to NED ==
  data: GoalLLA input; GoalNED output; NED_origin input
function GoalNED = LLA2NEDfun(GoalLLA,NED_origin)
%Written by Anderson Lebbad on September 20, 2014
%Last edited by:
%
%This function converts a target Latitude, Longitude, Altitude (LLA) point
%into North, East, Down (NED) coordinates
GoalNED = zeros(size(GoalLLA));
for i = 1:size(GoalLLA,1)
    %First convert to earth centered, earth fixed frame
    GoalECEF = lla2ecef([GoalLLA(1)*(pi/180), GoalLLA(2)*(pi/180), 0]');
    %Then convert from ECEF to North East Down
    GoalNEDvect = ecef2ned([NED_origin(1)*(pi/180),NED_origin(2)*(pi/180)],GoalECEF);
    GoalNED(i,:) = GoalNEDvect(1:2)';
end

end

function x_ecef = lla2ecef(x_lla)
% LLE2ECEF: Converts from geodetic latitude, longitude, and altitude to earth-centered earth-fixed Cartesian coordinates
% INPUT: latitude phi (rad), longitude lambda (rad), altitude h (m)
% OUTPUT: [x, y, z]' (m) earth-centered earth-fixed Cartesian coordinates
    a = 6378137; % equatorial radius of ellipsoid (semi-major axis) (m)
    b = 6356752; % polar axis radius of ellipsoid (semi-minor axis) (m)

    phi = x_lla(1);
    lambda = x_lla(2);
    h = x_lla(3);
    
    % auxiliar quantities f, e, and N
    f = (a-b)/a;
    e = f*(2-f);
    N = a/sqrt(1-(e*sin(phi))^2);
    x_ecef = [(N+h)*cos(phi)*cos(lambda); (N+h)*cos(phi)*sin(lambda); (N*(1-e^2)+h)*sin(phi)];
end

function [x_ned] = ecef2ned(ned_lla, x_ecef)
% ECEF2NED Converts from earth-centered, earth-fixed Cartesian coordinates to tangent plane
% INPUT:
% 1) x_ecef=[x,y,z]' (m) earth-centered, earth-fixed Cartesian coordinates
% 2) ned_lla=[phi,lambda]' consiting of latitude phi (rad), longitude lambda (rad) of NED origin
% OUTPUT:
% 1) x_ned=[x,y,z]' (m) in NED coordinate system with the origin [phi,lambda]'

    phi = ned_lla(1);
    lambda = ned_lla(2);

    % transformation  matrix
    T = [-sin(phi)*cos(lambda) -sin(phi)*sin(lambda)  cos(phi)
         -sin(lambda)           cos(lambda)           0
          cos(phi)*cos(lambda)   cos(phi)*sin(lambda)  sin(phi)];

     x_ned = T*(x_ecef-lla2ecef([phi, lambda, 0]')); % convert to NED
     x_ned(3) = -x_ned(3);
end

== matlab function RobotX_ss_acousticsSingle_Dock_LBskip_ODOA_T_1024_NewLidarMode/Main FSM/Docking/Docking/LLA to NED ==
  data: Course input; LLAs input; GoalNED output; NED_origin input
function GoalNED = LLA2NEDfun(Course,LLAs,NED_origin)
%Written by Anderson Lebbad on September 20, 2014
%Last edited by:
%
%This function converts a target Latitude, Longitude, Altitude (LLA) point
%into North, East, Down (NED) coordinates

NED  = zeros(4,2);
for i=1:4
%First convert to earth centered, earth fixed frame
GoalECEF = lla2ecef([LLAs(i,:)*(pi/180), 0]');
%Then convert from ECEF to North East Down
GoalNEDvect = ecef2ned(NED_origin'*(pi/180),GoalECEF);
NED(i,:) = GoalNEDvect(1:2)';
end

GoalNED = sum(NED)/4;

if Course == uint8('T')
    GoalNED = LLAs(1,:);
end

end

function x_ecef = lla2ecef(x_lla)
% LLE2ECEF: Converts from geodetic latitude, longitude, and altitude to earth-centered earth-fixed Cartesian coordinates
% INPUT: latitude phi (rad), longitude lambda (rad), altitude h (m)
% OUTPUT: [x, y, z]' (m) earth-centered earth-fixed Cartesian coordinates
    a = 6378137; % equatorial radius of ellipsoid (semi-major axis) (m)
    b = 6356752; % polar axis radius of ellipsoid (semi-minor axis) (m)

    phi = x_lla(1);
    lambda = x_lla(2);
    h = x_lla(3);
    
    % auxiliar quantities f, e, and N
    f = (a-b)/a;
    e = f*(2-f);
    N = a/sqrt(1-(e*sin(phi))^2);
    x_ecef = [(N+h)*cos(phi)*cos(lambda); (N+h)*cos(phi)*sin(lambda); (N*(1-e^2)+h)*sin(phi)];
end

function [x_ned] = ecef2ned(ned_lla, x_ecef)
% ECEF2NED Converts from earth-centered, earth-fixed Cartesian coordinates to tangent plane
% INPUT:
% 1) x_ecef=[x,y,z]' (m) earth-centered, earth-fixed Cartesian coordinates
% 2) ned_lla=[phi,lambda]' consiting of latitude phi (rad), longitude lambda (rad) of NED origin
% OUTPUT:
% 1) x_ned=[x,y,z]' (m) in NED coordinate system with the origin [phi,lambda]'

    phi = ned_lla(1);
    lambda = ned_lla(2);

    % transformation  matrix
    T = [-sin(phi)*cos(lambda) -sin(phi)*sin(lambda)  cos(phi)
         -sin(lambda)           cos(lambda)           0
          cos(phi)*cos(lambda)   cos(phi)*sin(lambda)  sin(phi)];

     x_ned = T*(x_ecef-lla2ecef([phi, lambda, 0]')); % convert to NED
     x_ned(3) = -x_ned(3);
end

== matlab function RobotX_ss_acousticsSingle_Dock_LBskip_ODOA_T_1024_NewLidarMode/Sensors/1020 Comms/Data Update1 ==
  data: Valid input; ControlMode input; V output; C output; L output; A output; Data input; D1 output; D2 output; D3 output; D4 output; D5 output; D6 output; D7 output; D8 output; D9 output; D10 output; D11 output; D12 output; D13 output; D14 output; D15 output; D16 output; D17 output; D18 output; D19 output; D20 output; D21 output; D22 output; D23 output; D24 output; Activate input
function [V,C,L,A,D1,D2,D3,D4,D5,D6,D7,D8,D9,D10,D11,D12,D13,D14,D15,D16,D17,...
    D18,D19,D20,D21,D22,D23,D24] = dataSplit(Valid,ControlMode,Data,Activate)
%Written by Anderson Lebbad on August 10, 2014
%Last Edited by: Anderson Lebbad on September 11, 2014

%This function splits the data vector into the twelve channels it is
%composed of for communication

persistent HoldData

A = Activate;

if isempty(HoldData)
    HoldData = zeros(26,1);
end

L = 8;

if Valid == 1
    HoldData(1) = Valid;
    HoldData(2) = ControlMode;
    HoldData(3) = Data(1);
    HoldData(4) = Data(2);
    HoldData(5) = Data(3);
    HoldData(6) = Data(4);
    HoldData(7) = Data(5);
    HoldData(8) = Data(6);
    HoldData(9) = Data(7);
    HoldData(10) = Data(8);
    HoldData(11) = Data(9);
    HoldData(12) = Data(10);
    HoldData(13) = Data(11);
    HoldData(14) = Data(12);
    HoldData(15) = Data(13);
    HoldData(16) = Data(14);
    HoldData(17) = Data(15);
    HoldData(18) = Data(16);
    HoldData(19) = Data(17);
    HoldData(20) = Data(18);
    HoldData(21) = Data(19);
    HoldData(22) = Data(20);
    HoldData(23) = Data(21);
    HoldData(24) = Data(22);
    HoldData(25) = Data(23);
    HoldData(26) = Data(24);
end

V = HoldData(1);
C = HoldData(2);
D1 = HoldData(3);
D2 = HoldData(4);
D3 = HoldData(5);
D4 = HoldData(6);
D5 = HoldData(7);
D6 = HoldData(8);
D7 = HoldData(9);
D8 = HoldData(10);
D9 = HoldData(11);
D10 = HoldData(12);
D11 = HoldData(13);
D12 = HoldData(14);
D13 = HoldData(15);
D14 = HoldData(16);
D15 = HoldData(17);
D16 = HoldData(18);
D17 = HoldData(19);
D18 = HoldData(20);
D19 = HoldData(21);
D20 = HoldData(22);
D21 = HoldData(23);
D22 = HoldData(24);
D23 = HoldData(25);
D24 = HoldData(26);

end

== matlab function RobotX_ss_acousticsSingle_Dock_LBskip_ODOA_T_1024_NewLidarMode/Sensors/1020 Comms/MATLAB Function2 ==
  data: Time input; asciiLIT output; Sequence input
% This function creates the light tower message to be sent from 
% Speedgoat in ascii code
% Written by: Edward Zhu
% Date: 9/17/14

function asciiLIT = asciiLITEncoder(Time, Sequence)

% Initialize output message vector as the serial output block expects 128
% character message
asciiLIT = uint8(zeros(1,128));

% Convert static strings to ascii code
asciiMsgID = uint8('$RXLIT,');
asciiComma = uint8(',');
asciiTeamID = uint8('FAUVU,');
asciiMsgEnd = uint8('*');
asciiMsgCRLF = [13 10];

% Convert UTC Time input (hhmmss) into ascii code
asciiTime = uint8(zeros(1,7));
asciiTime(7) = asciiComma;

for timeChar = 1:6
    asciiTime(timeChar) = floor(mod(Time,10^(7-timeChar))/...
        10^(6-timeChar)) + 48;
end

% Convert the light sequece into ascii code (1 = R, 2 = B, 3 = G)
asciiSeq = uint8(zeros(1,4)+32);
asciiSeq(4) = asciiMsgEnd;

if Sequence(1) > 0 && Sequence(2) > 0 && Sequence(3) > 0
    for seqChar = 1:3
        if Sequence(seqChar) == 1
            Sequence(seqChar) = uint8('R');
        elseif Sequence(seqChar) == 2
            Sequence(seqChar) = uint8('B');
        elseif Sequence(seqChar) == 3
            Sequence(seqChar) = uint8('G');
        end
    end
    asciiSeq(1:3) = Sequence;
end

% Concat individual ascii arrays into one array
asciiPreChkSum = cat(2,asciiMsgID,asciiTime,asciiTeamID,asciiSeq);

% Calculate the checksum of the message from the '$' to the '*' and convert
% to hex
chkSum = uint8(0);

for chksumChar = 1:(length(asciiPreChkSum)-2)
    chkSum = bitxor(chkSum,asciiPreChkSum(chksumChar+1));
end

% Convert the checksum to ascii
chkSum = dec2hex(chkSum);
asciiChkSum = uint8(zeros(1,length(chkSum))+32);
for i = 1:length(chkSum)
    asciiChkSum(i) = uint8(chkSum(i));
end

% Concat the checksum and the '/r/n' to the end of the message
asciiPostChkSum = cat(2,asciiPreChkSum,asciiChkSum,asciiMsgCRLF);

% Output the final message
asciiLIT(1:length(asciiPostChkSum)) = asciiPostChkSum;

== matlab function RobotX_ss_acousticsSingle_Dock_LBskip_ODOA_T_1024_NewLidarMode/Main FSM/LightTower/Sweep Field/Spin, Listen, and Point/Look for Light Tower ==
  data: subsetCorners input; X input; Y input; Psi input; Distances input; Angles input; Data output; Finished output; FoundTower output; TowerLoc output; spinAmount input
function [Data, Finished, FoundTower, TowerLoc] = fcn(...
    subsetCorners, X, Y, Psi, Distances, Angles, spinAmount)

%   Written by Michael Benson on October 23, 2014
%   This function spins the WAM-V to look for the light tower.  If it
%   sees an object, and that object is within the field subset, the boat
%   will hold pose and the Lidar will continue to evaluate an object.  If
%   the object is still there within that time, it determines that that
%   object is the buoy and ends the task.  Otherwise, the task exits
%   without setting FoundTower high.

[Distances,I] = sort(Distances);
Angles = Angles(I);

persistent FoundHeading FoundCounter desiredHeading initHeading minPose maxPose minReached maxReached

offset = 5;

if isempty(FoundHeading) && isempty(FoundCounter) && isempty(desiredHeading) && isempty(initHeading) && isempty(minReached) && isempty(maxReached)
    FoundCounter = 0;
    minPose = Psi - spinAmount/2;
    maxPose = Psi + spinAmount/2;
    minReached = 0;
    maxReached = 0;
    initHeading = Psi;
    desiredHeading = Psi+offset;
    FoundHeading = 0;
end

Finished = 0;
FoundTower = 0;
Data = zeros(24,1);
TowerLoc = zeros(1,2);
LandmarkLocations = zeros(12,2);
LandmarkDistances = zeros(12,1);

ObjectInfo = [Distances,Angles];


%% Landmark Analysis
if ObjectInfo(12,1) ~= 0 && ObjectInfo(12,2) ~= 0
    %calculate location of each landmark and determine if it is in the
    %bounding box
    for i = 12-sum(Distances ~= 0)+1:12
        LandmarkX = X + cos((Psi+Angles(i))*pi/180)*Distances(i)/100;
        LandmarkY = Y + sin((Psi+Angles(i))*pi/180)*Distances(i)/100;
        LandmarkValid = inBbox(subsetCorners,[LandmarkX LandmarkY]);
        if LandmarkValid == 1
            LandmarkLocations(i,1:2) = [LandmarkX LandmarkY];
            LandmarkDistances(i) = Distances(i);
        end
    end
    
    [~,I] = sort(LandmarkDistances);
    LandmarkLocations = LandmarkLocations(I);
    
    if sum(LandmarkDistances ~= 0) >= 1
        FoundTower = 1;
        TowerLoc = LandmarkLocations(12-sum(LandmarkDistances ~= 0)+1,1:2);
        FoundCounter = FoundCounter + 1;
        if FoundCounter == 1;
            FoundHeading = Psi;
        end
        desiredHeading = FoundHeading;
    end
else
    FoundCounter = 0;
    if abs(Psi-maxPose) < 5
        maxReached = 1;
    elseif abs(Psi-minPose) < 5
        minReached = 1;
    end
    
    if maxReached == 1
        desiredHeading = Psi - offset;
    elseif maxReached == 1 && minReached == 1
        desiredHeading = initHeading;
        Finished = 1;
    end
end

Data(1:3) = [X Y desiredHeading];

end

function [ inBbox ] = inBbox( bbox, point )
%UNTITLED Summary of this function goes here
%   Detailed explanation goes here
b1 = bbox(1,:);
b2 = bbox(2,:);
b3 = bbox(3,:);
b4 = bbox(4,:);

t1 = inTriangle(point,b1,b2,b3);
t2 = inTriangle(point,b1,b2,b4);
t3 = inTriangle(point,b1,b3,b4);

if t1 && t2 && t3
    inBbox = 1;
else
    inBbox = 0;
end

end

function [ inTri ] = inTriangle(p, a, b, c)

s1 = sameSide(p,a,b,c);
s2 = sameSide(p,b,a,c);
s3 = sameSide(p,c,a,b);

if s1 || s2 || s3
    inTri = 1;
else
    inTri = 0;
end

end

function [ onSame ] = sameSide(p1,p2,a,b)

theta = atan2(b(2)-a(2),b(1)-a(1));
R = [cos(theta), sin(theta); -sin(theta), cos(theta)];
side1 = R*(p1-a)';
side2 = R*(p2-a)';
same = side1(2)/side2(2);
onSame = same >= 0;

end

== matlab function RobotX_ss_acousticsSingle_Dock_LBskip_ODOA_T_1024_NewLidarMode/Main FSM/LightTower/Turn For Sweep/LLA to NED ==
  data: GoalLLA input; GoalNED output; NED_origin input
function GoalNED = LLA2NEDfun(GoalLLA,NED_origin)
%Written by Anderson Lebbad on September 20, 2014
%Last edited by:
%
%This function converts a target Latitude, Longitude, Altitude (LLA) point
%into North, East, Down (NED) coordinates
GoalNED = zeros(size(GoalLLA));
for i = 1:size(GoalLLA,1)
    %First convert to earth centered, earth fixed frame
    GoalECEF = lla2ecef([GoalLLA(1)*(pi/180), GoalLLA(2)*(pi/180), 0]');
    %Then convert from ECEF to North East Down
    GoalNEDvect = ecef2ned([NED_origin(1)*(pi/180),NED_origin(2)*(pi/180)],GoalECEF);
    GoalNED(i,:) = GoalNEDvect(1:2)';
end

end

function x_ecef = lla2ecef(x_lla)
% LLE2ECEF: Converts from geodetic latitude, longitude, and altitude to earth-centered earth-fixed Cartesian coordinates
% INPUT: latitude phi (rad), longitude lambda (rad), altitude h (m)
% OUTPUT: [x, y, z]' (m) earth-centered earth-fixed Cartesian coordinates
    a = 6378137; % equatorial radius of ellipsoid (semi-major axis) (m)
    b = 6356752; % polar axis radius of ellipsoid (semi-minor axis) (m)

    phi = x_lla(1);
    lambda = x_lla(2);
    h = x_lla(3);
    
    % auxiliar quantities f, e, and N
    f = (a-b)/a;
    e = f*(2-f);
    N = a/sqrt(1-(e*sin(phi))^2);
    x_ecef = [(N+h)*cos(phi)*cos(lambda); (N+h)*cos(phi)*sin(lambda); (N*(1-e^2)+h)*sin(phi)];
end

function [x_ned] = ecef2ned(ned_lla, x_ecef)
% ECEF2NED Converts from earth-centered, earth-fixed Cartesian coordinates to tangent plane
% INPUT:
% 1) x_ecef=[x,y,z]' (m) earth-centered, earth-fixed Cartesian coordinates
% 2) ned_lla=[phi,lambda]' consiting of latitude phi (rad), longitude lambda (rad) of NED origin
% OUTPUT:
% 1) x_ned=[x,y,z]' (m) in NED coordinate system with the origin [phi,lambda]'

    phi = ned_lla(1);
    lambda = ned_lla(2);

    % transformation  matrix
    T = [-sin(phi)*cos(lambda) -sin(phi)*sin(lambda)  cos(phi)
         -sin(lambda)           cos(lambda)           0
          cos(phi)*cos(lambda)   cos(phi)*sin(lambda)  sin(phi)];

     x_ned = T*(x_ecef-lla2ecef([phi, lambda, 0]')); % convert to NED
     x_ned(3) = -x_ned(3);
end

== matlab function RobotX_ss_acousticsSingle_Dock_LBskip_ODOA_T_1024_NewLidarMode/Main FSM/ODOA/Entry Gate/Entry Gate Align/MATLAB Function1 ==
  data: EnterGateNED input; entryNED output; gateNumber input
function entryNED = EntryGPSSelector(EnterGateNED,gateNumber)

entryNED = EnterGateNED(gateNumber,:);

== matlab function RobotX_ss_acousticsSingle_Dock_LBskip_ODOA_T_1024_NewLidarMode/Main FSM/ODOA/Entry Gate/Entry Gate Enabler ==
  data: StartFin input; TaskSelector output; StartEn output; AlignFin input; AlignEn output; ThroughEn output
function [TaskSelector, StartEn,AlignEn,ThroughEn] = entryGateEnabler(StartFin, AlignFin)

StartEn = 0;
AlignEn = 0;
ThroughEn = 0;

if StartFin == 0
    StartEn = 1;
    TaskSelector = 1;
elseif AlignFin == 0
    AlignEn = 1;
    TaskSelector = 2;
else
    ThroughEn = 1;
    TaskSelector = 3;
end

== matlab function RobotX_ss_acousticsSingle_Dock_LBskip_ODOA_T_1024_NewLidarMode/Main FSM/ODOA/Entry Gate/Entry Gate Through/CalcTimes ==
  data: pts input; u input; Data output
function Data = calcTimes(pts, u)
%Written by Anderson Lebbad on August 9, 2014
%Last Edited: Dylan DeGaetano September 1, 2014

%Calculates times for the boat to get to points for a trajectory, and
%formats Data for communication

%Initialize
Data = zeros(24,1);
traj = zeros(8,3);
traj(:,1:2) = pts;



for k = 2:8
    %Calculate distance to travel from last point
    distTravel = sqrt(sum((pts(k-1,:)-pts(k,:)).^2));
    %Assume 1m per second speed
    traj(k,3) = traj(k-1,3) + distTravel;
    %Add time based off initial velocity to get to first point past initial
    if k == 2
        traj(k,3) = traj(k,3) + 2.5*abs(2-u);
    end
end


%Output Data
for i=1:8
    for j = 1:3
        Data(3*(i-1)+j) = traj(i,j);
    end
end

== matlab function RobotX_ss_acousticsSingle_Dock_LBskip_ODOA_T_1024_NewLidarMode/Main FSM/ODOA/Entry Gate/Entry Gate Through/MATLAB Function ==
  data: dist input; X input; Y input; Psi input; GoalNED output
function GoalNED = travelAlongHeading(dist, X, Y, Psi)
%Written by Michael Benson on October 23, 2014

%This function determines the target NED point for the Sweep Field subtask
%for the Light Tower task.  The target point is Distance meters from the
%current ASV position, and is towards the opposite corner of the subset
%field.

persistent lockedHeading

Psi = Psi*180/pi;

if isempty(lockedHeading)
    lockedHeading = Psi;
end

GoalNED = [X+dist*cos(lockedHeading*pi/180) Y+dist*sin(lockedHeading*pi/180)];

== matlab function RobotX_ss_acousticsSingle_Dock_LBskip_ODOA_T_1024_NewLidarMode/Main FSM/ODOA/Entry Gate/GPS Move/GPSMove ==
  data: GoalNED input; X input; Finished output; valid output; Y input; Psi input; pts output
function [Finished,valid,pts] = GPSmove(GoalNED,X,Y,Psi)
%Written by Dylan DeGaetano on September 1, 2014
%Last edited by: Anderson Lebbad
%
%This function will go to a given NED cooridnate, last edit changed the
%goal pt and variable names

% Input of GoalNED is a 10x2 matrix of NED coords where the first row is
% the coord of the docking observation point

persistent Sample
if isempty(Sample)
Sample = 0;
end
Finished = 0;
pts = zeros(8,2);
%$Distance to object in meters
if Sample == 100
    Sample = 0;
end

if Sample == 0
    pts(1,1) = X+5*cos(Psi*pi/180);
    pts(1,2) = Y+5*sin(Psi*pi/180);
    pts(8,1) = GoalNED(1,1);
    pts(8,2) = GoalNED(1,2);
    pts(2,:) = pts(1,:) +(1*(GoalNED(1,:)-pts(1,:))/7);
    pts(3,:) = pts(1,:) +(2*(GoalNED(1,:)-pts(1,:))/7);
    pts(4,:) = pts(1,:) +(3*(GoalNED(1,:)-pts(1,:))/7);
    pts(5,:) = pts(1,:) +(4*(GoalNED(1,:)-pts(1,:))/7);
    pts(6,:) = pts(1,:) +(5*(GoalNED(1,:)-pts(1,:))/7);
    pts(7,:) = pts(1,:) +(6*(GoalNED(1,:)-pts(1,:))/7);
    Sample = 1; 
    valid = 1;
    
else 
    range = sqrt(sum((GoalNED(1,:) - [X Y]).^2));
    if range <= 5
        Finished = 1;
    end
    valid = 0;
    Sample = Sample + 1;
end

== matlab function RobotX_ss_acousticsSingle_Dock_LBskip_ODOA_T_1024_NewLidarMode/Main FSM/ODOA/Exit Gate/Exit Gate Through/MATLAB Function ==
  data: dist input; X input; Y input; Psi input; GoalNED output
function GoalNED = travelAlongHeading(dist, X, Y, Psi)
%Written by Michael Benson on October 23, 2014

%This function determines the target NED point for the Sweep Field subtask
%for the Light Tower task.  The target point is Distance meters from the
%current ASV position, and is towards the opposite corner of the subset
%field.

persistent lockedHeading

Psi = Psi*180/pi;

if isempty(lockedHeading)
    lockedHeading = Psi;
end

GoalNED = [X+dist*cos(lockedHeading*pi/180) Y+dist*sin(lockedHeading*pi/180)];

== matlab function RobotX_ss_acousticsSingle_Dock_LBskip_ODOA_T_1024_NewLidarMode/Main FSM/ODOA/GPS Beeline/MATLAB Function1 ==
  data: ExitGateGPS input; exitGPS output; gateNumber input
function exitGPS = ExitGPSSelector(ExitGateGPS,gateNumber)

exitGPS = [ExitGateGPS(gateNumber,1)+5,ExitGateGPS(gateNumber,2)];

== matlab function RobotX_ss_acousticsSingle_Dock_LBskip_ODOA_T_1024_NewLidarMode/Main FSM/ODOA/Obstacle Navigation Enabler ==
  data: enterGateFin input; dodgeIncomplete input; GPSBeeFin input; dodgeStart input; taskSelector output; entryGateEn output; dodgeEn output; GPSEn output; exitGateEn output
function [taskSelector, entryGateEn, dodgeEn, GPSEn, exitGateEn]  = obstNavEnabler(enterGateFin, dodgeIncomplete, GPSBeeFin, dodgeStart)

entryGateEn = 0;
GPSEn = 0;
dodgeEn = 0;
exitGateEn = 0;

if  enterGateFin == 0
    entryGateEn = 1;
    taskSelector = 1;
elseif dodgeStart == 1 || dodgeIncomplete == 1
    dodgeEn = 1;
    taskSelector = 2;
elseif GPSBeeFin == 1
    exitGateEn = 1;
    taskSelector = 3;
else
    GPSEn = 1;
    taskSelector = 4;
end

== matlab function RobotX_ss_acousticsSingle_Dock_LBskip_ODOA_T_1024_NewLidarMode/Main FSM/Start//Speedgate/Dead Reckon/Calculate Times ==
  data: pts input; u input; Data output
function Data = calcTimes(pts, u)
%Written by Anderson Lebbad on August 9, 2014
%Last Edited:

%Calculates times for the boat to get to points for a trajectory, and
%formats Data for communication

%Initialize
Data = zeros(24,1);
traj = zeros(8,3);

traj(:,1:2) = pts;

for k = 2:8
    %Calculate distance to travel from last point
    distTravel = sqrt(sum((pts(k-1,:)-pts(k,:)).^2));
    %Assume 1m per second speed
    traj(k,3) = traj(k-1,3) + distTravel;
    %Add time based off initial velocity to get to first point past initial
    if k == 2
        traj(k,3) = traj(k,3) + 2.5*abs(2-u);
    end
end


%Output Data
for i=1:8
    for j = 1:3
        Data(3*(i-1)+j) = traj(i,j);
    end
end
